simulink model "ex1_sim"  (R2014b)
settings: Solver=ode45  StartTime=0.0  StopTime=2  RelTol=1e-3
values from neighbouring files (symbols this model uses):
  d = 0.5    [ex1.m]
  freq = 10    [ex1.m]
  m = 0.1    [ex1.m]
settings Model: Creator=gabras  LastModifiedBy=gabras

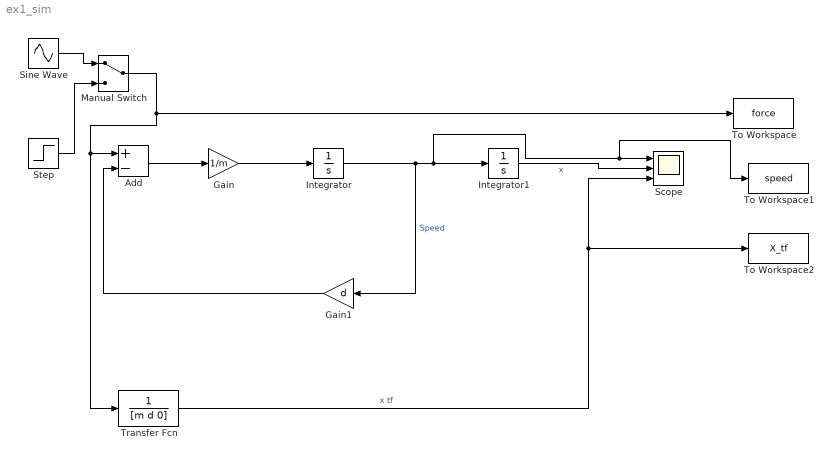
== system ex1_sim ==
  Add : Sum  Inputs=+-
  Gain : Gain  Gain=1/m
  Gain1 : Gain  Gain=d
  Integrator : Integrator
  Integrator1 : Integrator
  Manual Switch : ManualSwitch
  Scope : Scope  NumInputPorts=3
      settings: YMin=-5~-5~-5  YMax=5~5~5
  Sine Wave : Sin  Frequency=freq  SampleTime=0
  Step : Step  SampleTime=0
  To Workspace : ToWorkspace  VariableName=force  SaveFormat=Timeseries  SampleTime=-1
  To Workspace1 : ToWorkspace  VariableName=speed  SaveFormat=Timeseries  SampleTime=-1
  To Workspace2 : ToWorkspace  VariableName=X_tf  SaveFormat=Timeseries  SampleTime=-1
  Transfer Fcn : TransferFcn  Denominator=[m d 0]
  wires:
  Integrator/1 -> Gain1/1, To Workspace1/1, Scope/1, Integrator1/1  "Speed"
  Gain/1 -> Integrator/1
  Add/1 -> Gain/1
  Integrator1/1 -> Scope/2  "x"
  Gain1/1 -> Add/2
  Step/1 -> Manual Switch/2
  Transfer Fcn/1 -> Scope/3, To Workspace2/1  "x tf"
  Sine Wave/1 -> Manual Switch/1
  Manual Switch/1 -> To Workspace/1, Transfer Fcn/1, Add/1
